simulink model "Simul_Trab2"  (R2019a)
settings: Solver=VariableStepAuto  StartTime=0.0  StopTime=10  RelTol=1e-3
settings Model: Creator=erica  LastModifiedBy=erica

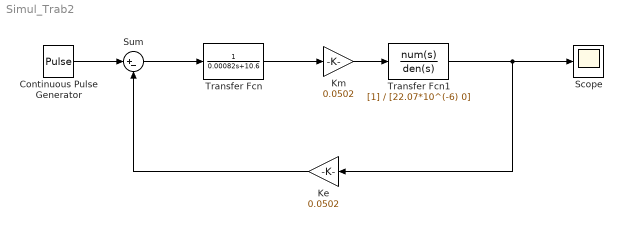
== system Simul_Trab2 ==
  Continuous Pulse Generator : DiscretePulseGenerator  PulseType=Time based  Amplitude=5  Period=1  PulseWidth=50
  Ke : Gain  Gain=0.0502
  "Km " : Gain  Gain=0.0502
  Scope : Scope
  Sum : Sum  Inputs=|+-
  Transfer Fcn : TransferFcn  Denominator=[0.00082 10.6]
  Transfer Fcn1 : TransferFcn  Denominator=[22.07*10^(-6) 0]
  wires:
  Transfer Fcn/1 -> "Km "/1
  "Km "/1 -> Transfer Fcn1/1
  Transfer Fcn1/1 -> Ke/1, Scope/1
  Continuous Pulse Generator/1 -> Sum/1
  Sum/1 -> Transfer Fcn/1
  Ke/1 -> Sum/2
